simulink model "c_lab3_3sim"  (R2020b)
settings: Solver=VariableStepAuto  StartTime=0.0  StopTime=150  RelTol=1e-3
settings Model: Creator=musa oğural  LastModifiedBy=musa oğural

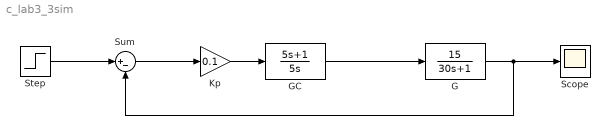
== system c_lab3_3sim ==
  G : TransferFcn  Numerator=[15]  Denominator=[30 1]
  GC : TransferFcn  Numerator=[5 1]  Denominator=[5 0]
  Kp : Gain  Gain=0.1
  Scope : Scope
  Step : Step  Time=0  SampleTime=0
  Sum : Sum  Inputs=|+-
  wires:
  Step/1 -> Sum/1
  Sum/1 -> Kp/1
  Kp/1 -> GC/1
  GC/1 -> G/1
  G/1 -> Scope/1, Sum/2
